simulink model "plant_examples"  (R2023b)
settings: Solver=VariableStepAuto  StartTime=0.0  StopTime=10.0  RelTol=1e-3
undefined symbols (not defined in the file or in its folder): param, x0
libraries: fl_lib x40, nesl_utility x18, simulink x8
(part 3 of 3)

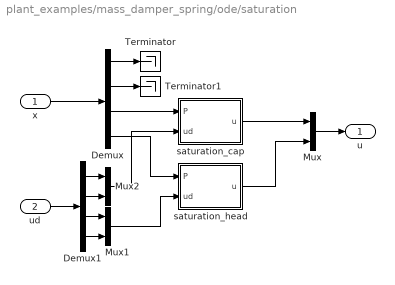
== system plant_examples/mass_damper_spring/ode/saturation ==
  x : Inport  PortDimensions=param.xdim
  ud : Inport  Port=2  PortDimensions=param.udim
  Demux : Demux
  Demux1 : Demux
  Mux : Mux  Inputs=2
  Mux1 : Mux  Inputs=2
  Mux2 : Mux  Inputs=2
  Terminator : Terminator
  Terminator1 : Terminator
  saturation_cap : Subsystem
  saturation_head : Subsystem
  u : Outport
  wires:
  x/1 -> Demux/1
  Demux/3 -> saturation_cap/1(P)
  Demux/4 -> saturation_head/1(P)
  Demux/1 -> Terminator/1
  Demux/2 -> Terminator1/1
  saturation_cap/1(u) -> Mux/1
  saturation_head/1(u) -> Mux/2
  Mux/1 -> u/1
  ud/1 -> Demux1/1
  Demux1/4 -> Mux1/2
  Demux1/3 -> Mux1/1
  Demux1/1 -> Mux2/1
  Demux1/2 -> Mux2/2
  Mux2/1 -> saturation_cap/2(ud)
  Mux1/1 -> saturation_head/2(ud)

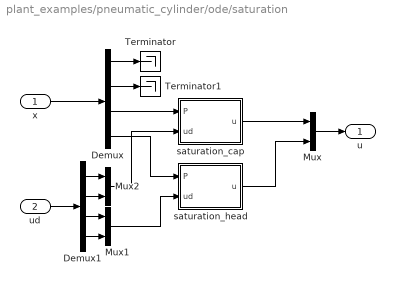
== system plant_examples/pneumatic_cylinder/ode/saturation ==
  x : Inport  PortDimensions=param.xdim
  ud : Inport  Port=2  PortDimensions=param.udim
  Demux : Demux
  Demux1 : Demux
  Mux : Mux  Inputs=2
  Mux1 : Mux  Inputs=2
  Mux2 : Mux  Inputs=2
  Terminator : Terminator
  Terminator1 : Terminator
  saturation_cap : Subsystem
  saturation_head : Subsystem
  u : Outport
  wires:
  x/1 -> Demux/1
  Demux/3 -> saturation_cap/1(P)
  Demux/4 -> saturation_head/1(P)
  Demux/1 -> Terminator/1
  Demux/2 -> Terminator1/1
  saturation_cap/1(u) -> Mux/1
  saturation_head/1(u) -> Mux/2
  Mux/1 -> u/1
  ud/1 -> Demux1/1
  Demux1/4 -> Mux1/2
  Demux1/3 -> Mux1/1
  Demux1/1 -> Mux2/1
  Demux1/2 -> Mux2/2
  Mux2/1 -> saturation_cap/2(ud)
  Mux1/1 -> saturation_head/2(ud)

== system plant_examples/pneumatic_cylinder/simscape/Vctube ==
  Ta : fl_lib/Thermal/Thermal Sources/Temperature Source  temperature=param.Ta K
  Vctube : fl_lib/Gas/Elements/Constant Volume Chamber (G)  volume=param.Vctube m^3  num_ports=foundation.enum.num_ports.one  area_A=0.01 m^2  area_B=0.01 m^2  area_C=0.01 m^2  area_D=0.01 m^2  p_I_specify=on  p_I_priority=High  p_I=x0(3) Pa  p_I_nominal_specify=off  p_I_nominal_unit=MPa  p_I_nominal_value=1  T_I_specify=off  T_I_priority=High  T_I=293.15 K  T_I_nominal_specify=off  T_I_nominal_unit=K  T_I_nominal_value=1  rho_I_specify=off  rho_I_priority=None  rho_I=1.2 kg/m^3  rho_I_nominal_specify=off  rho_I_nominal_unit=kg/m^3  rho_I_nominal_value=1
      settings: InternalSimscapePortConfiguration="{\"Bottom\":[],\"Left\":[{\"id\":\"A\",\"label\":\"A\",\"type\":\"foundation.gas.gas\"},{\"id\":\"H\",\"label\":\"H\",\"type\":\"foundation.thermal.thermal\"}],\"Right\":[],\"Top\":[]}"
  A : PMIOPort  Side=Left
  B : PMIOPort  Port=2  Side=Right
  connections:
  A/RConn1 -- B/RConn1 -- Vctube/LConn1
  Ta/LConn1 -- Vctube/LConn2

== system plant_examples/pneumatic_cylinder/simscape/Vhtube ==
  Ta : fl_lib/Thermal/Thermal Sources/Temperature Source  temperature=param.Ta K
  Vhtube : fl_lib/Gas/Elements/Constant Volume Chamber (G)  volume=param.Vhtube m^3  num_ports=foundation.enum.num_ports.one  area_A=0.01 m^2  area_B=0.01 m^2  area_C=0.01 m^2  area_D=0.01 m^2  p_I_specify=on  p_I_priority=High  p_I=x0(4) Pa  p_I_nominal_specify=off  p_I_nominal_unit=MPa  p_I_nominal_value=1  T_I_specify=off  T_I_priority=High  T_I=293.15 K  T_I_nominal_specify=off  T_I_nominal_unit=K  T_I_nominal_value=1  rho_I_specify=off  rho_I_priority=None  rho_I=1.2 kg/m^3  rho_I_nominal_specify=off  rho_I_nominal_unit=kg/m^3  rho_I_nominal_value=1
      settings: InternalSimscapePortConfiguration="{\"Bottom\":[],\"Left\":[{\"id\":\"A\",\"label\":\"A\",\"type\":\"foundation.gas.gas\"},{\"id\":\"H\",\"label\":\"H\",\"type\":\"foundation.thermal.thermal\"}],\"Right\":[],\"Top\":[]}"
  A : PMIOPort  Side=Left
  B : PMIOPort  Port=2  Side=Right
  connections:
  A/RConn1 -- Vhtube/LConn1 -- B/RConn1
  Ta/LConn1 -- Vhtube/LConn2

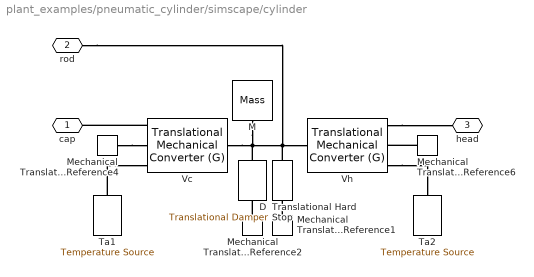
== system plant_examples/pneumatic_cylinder/simscape/cylinder ==
  D : fl_lib/Mechanical/Translational Elements/Translational Damper  D=param.D N*s/m  v_specify=off  v_priority=None  v=0 m/s  v_nominal_specify=off  v_nominal_unit=m/s  v_nominal_value=1  f_specify=off  f_priority=None  f=0 N  f_nominal_specify=off  f_nominal_unit=N  f_nominal_value=1
  M : fl_lib/Mechanical/Translational Elements/Mass  mass=param.M kg  num_ports=foundation.enum.numPorts2.one  v_specify=off  v_priority=High  v=0 m/s  v_nominal_specify=off  v_nominal_unit=m/s  v_nominal_value=1  f_specify=off  f_priority=None  f=0 N  f_nominal_specify=off  f_nominal_unit=N  f_nominal_value=1
  Mechanical Translational Reference{1..2,4,6} (4 alike) : fl_lib/Mechanical/Translational Elements/Mechanical Translational Reference
  Ta1 : fl_lib/Thermal/Thermal Sources/Temperature Source  temperature=param.Ta K
  Ta2 : fl_lib/Thermal/Thermal Sources/Temperature Source  temperature=param.Ta K
  Translational Hard Stop : fl_lib/Mechanical/Translational Elements/Translational Hard Stop  upper_bnd=0.5*param.L m  lower_bnd=-0.5*param.L m  model=simscape.enum.hardstop.fulldamped  stiff_up=1e6 N/m  stiff_low=1e6 N/m  D_up=150 N*s/m  D_low=150 N*s/m  transition=0.1 mm  coeff_rest=0.7  v_tol=0.001 m/s  f_tol=0.001 N  v_specify=off  v_priority=None  v=0 m/s  v_nominal_specify=off  v_nominal_unit=m/s  v_nominal_value=1  f_specify=off  f_priority=None  f=0 N  f_nominal_specify=off  f_nominal_unit=N  f_nominal_value=1  x_specify=on  x_priority=High  x=x0(1) m  x_nominal_specify=off  x_nominal_unit=m  x_nominal_value=1  M_specify=off  M_priority=None  M=0
  Vc : fl_lib/Gas/Elements/Translational Mechanical Converter (G)  mech_orientation=foundation.enum.MechOrientationTranslational.Positive  displacement_spec=foundation.enum.DisplacementSpec.Calculate  length_init=x0(1)+0.5*param.L m  interface_area=param.Ac m^2  dead_volume=param.Vc0 m^3  area_A=0.01 m^2  environment_spec=foundation.enum.pressure_spec.atmospheric  environment_pressure=0.101325 MPa  p_I_specify=on  p_I_priority=High  p_I=x0(3) Pa  p_I_nominal_specify=off  p_I_nominal_unit=MPa  p_I_nominal_value=1  T_I_specify=off  T_I_priority=High  T_I=293.15 K  T_I_nominal_specify=off  T_I_nominal_unit=K  T_I_nominal_value=1  rho_I_specify=off  rho_I_priority=None  rho_I=1.2 kg/m^3  rho_I_nominal_specify=off  rho_I_nominal_unit=kg/m^3  rho_I_nominal_value=1
      settings: InternalSimscapePortConfiguration="{\"Bottom\":[],\"Left\":[{\"id\":\"A\",\"label\":\"A\",\"type\":\"foundation.gas.gas\"},{\"id\":\"C\",\"label\":\"C\",\"type\":\"foundation.mechanical.translational.translational\"},{\"id\":\"H\",\"label\":\"H\",\"type\":\"foundation.thermal.thermal\"}],\"Right\":[{\"id\":\"R\",\"label\":\"R\",\"type\":\"foundation.mechanical.translational.translational\"}],\"Top\":[]}"
  Vh : fl_lib/Gas/Elements/Translational Mechanical Converter (G)  mech_orientation=foundation.enum.MechOrientationTranslational.Negative  displacement_spec=foundation.enum.DisplacementSpec.Calculate  length_init=x0(1)-0.5*param.L m  interface_area=param.Ah m^2  dead_volume=param.Vh0 m^3  area_A=0.01 m^2  environment_spec=foundation.enum.pressure_spec.atmospheric  environment_pressure=0.101325 MPa  p_I_specify=on  p_I_priority=High  p_I=x0(4) Pa  p_I_nominal_specify=off  p_I_nominal_unit=MPa  p_I_nominal_value=1  T_I_specify=off  T_I_priority=High  T_I=293.15 K  T_I_nominal_specify=off  T_I_nominal_unit=K  T_I_nominal_value=1  rho_I_specify=off  rho_I_priority=None  rho_I=1.2 kg/m^3  rho_I_nominal_specify=off  rho_I_nominal_unit=kg/m^3  rho_I_nominal_value=1
      settings: InternalSimscapePortConfiguration="{\"Bottom\":[],\"Left\":[{\"id\":\"A\",\"label\":\"A\",\"type\":\"foundation.gas.gas\"},{\"id\":\"C\",\"label\":\"C\",\"type\":\"foundation.mechanical.translational.translational\"},{\"id\":\"H\",\"label\":\"H\",\"type\":\"foundation.thermal.thermal\"}],\"Right\":[{\"id\":\"R\",\"label\":\"R\",\"type\":\"foundation.mechanical.translational.translational\"}],\"Top\":[]}"
  cap : PMIOPort  Side=Left
  rod : PMIOPort  Port=2  Side=Left
  head : PMIOPort  Port=3  Side=Right
  connections:
  Mechanical Translational Reference4/LConn1 -- Vc/LConn2
  Mechanical Translational Reference6/LConn1 -- Vh/LConn2
  Vh/LConn1 -- head/RConn1
  Mechanical Translational Reference2/LConn1 -- D/RConn1
  Vc/RConn1 -- rod/RConn1 -- Translational Hard Stop/LConn1 -- Vh/RConn1 -- M/LConn1 -- D/LConn1
  Mechanical Translational Reference1/LConn1 -- Translational Hard Stop/RConn1
  Vc/LConn1 -- cap/RConn1
  Ta1/LConn1 -- Vc/LConn3
  Vh/LConn3 -- Ta2/LConn1

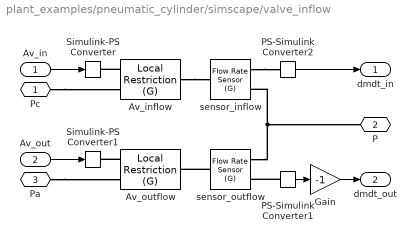
== system plant_examples/pneumatic_cylinder/simscape/valve_inflow ==
  Av_in : Inport
  Av_out : Inport  Port=2
  Av_inflow : fl_lib/Gas/Elements/Local Restriction (G)  restriction_type=foundation.enum.restriction_type.variable  restriction_area=1e-3 m^2  min_area=eps m^2  max_area=param.Av m^2  area=0.01 m^2  Cd=0.8975  B_lam=0.999
      settings: InternalSimscapePortConfiguration="{\"Bottom\":[],\"Left\":[{\"id\":\"A\",\"label\":\"A\",\"type\":\"foundation.gas.gas\"},{\"id\":\"area_in\",\"label\":\"AR\",\"type\":\"input\"}],\"Right\":[{\"id\":\"B\",\"label\":\"B\",\"type\":\"foundation.gas.gas\"}],\"Top\":[]}"
  Av_outflow : fl_lib/Gas/Elements/Local Restriction (G)  restriction_type=foundation.enum.restriction_type.variable  restriction_area=1e-3 m^2  min_area=eps m^2  max_area=param.Av m^2  area=0.01 m^2  Cd=0.8975  B_lam=0.999
      settings: InternalSimscapePortConfiguration="{\"Bottom\":[],\"Left\":[{\"id\":\"A\",\"label\":\"A\",\"type\":\"foundation.gas.gas\"},{\"id\":\"area_in\",\"label\":\"AR\",\"type\":\"input\"}],\"Right\":[{\"id\":\"B\",\"label\":\"B\",\"type\":\"foundation.gas.gas\"}],\"Top\":[]}"
  Gain : Gain  Gain=-1
  PS-Simulink Converter1 : nesl_utility/PS-Simulink Converter  PhysicalDomain=network_engine_domain  SubClassName=ps_output  LeftPortType=input  RightPortType=output  PseudoPeriodic=off  Frequencies=[]  VectorFormat=inherit  Unit=inherit  AffineConversion=off
  PS-Simulink Converter2 : nesl_utility/PS-Simulink Converter  PhysicalDomain=network_engine_domain  SubClassName=ps_output  LeftPortType=input  RightPortType=output  PseudoPeriodic=off  Frequencies=[]  VectorFormat=inherit  Unit=inherit  AffineConversion=off
  Simulink-PS Converter : nesl_utility/Simulink-PS Converter  PhysicalDomain=network_engine_domain  SubClassName=ps_input  LeftPortType=input  RightPortType=output  PseudoPeriodic=off  Frequencies=[]  NoiseDistribution=none  NoiseParameters=[]  Unit=1  AffineConversion=off  FilteringAndDerivatives=provide  SimscapeFilterOrder=1  InputFilterTimeConstant=0.001  UdotUserProvided=0
  Simulink-PS Converter1 : nesl_utility/Simulink-PS Converter  PhysicalDomain=network_engine_domain  SubClassName=ps_input  LeftPortType=input  RightPortType=output  PseudoPeriodic=off  Frequencies=[]  NoiseDistribution=none  NoiseParameters=[]  Unit=1  AffineConversion=off  FilteringAndDerivatives=provide  SimscapeFilterOrder=1  InputFilterTimeConstant=0.001  UdotUserProvided=0
  sensor_inflow : fl_lib/Gas/Sensors/Flow Rate Sensor (G)  mass_flow_measure=true  volumetric_flow_measure=false  volumetric_flow_conditions=foundation.enum.volumetric_flow_conditions.actual  p_std=0.101325 MPa  T_std=20 degC  energy_flow_measure=false
      settings: InternalSimscapePortConfiguration="{\"Bottom\":[],\"Left\":[{\"id\":\"A\",\"label\":\"A\",\"type\":\"foundation.gas.gas\"}],\"Right\":[{\"id\":\"B\",\"label\":\"B\",\"type\":\"foundation.gas.gas\"},{\"id\":\"M\",\"label\":\"M\",\"type\":\"output\"}],\"Top\":[]}"
  sensor_outflow : fl_lib/Gas/Sensors/Flow Rate Sensor (G)  mass_flow_measure=true  volumetric_flow_measure=false  volumetric_flow_conditions=foundation.enum.volumetric_flow_conditions.actual  p_std=0.101325 MPa  T_std=20 degC  energy_flow_measure=false
      settings: InternalSimscapePortConfiguration="{\"Bottom\":[],\"Left\":[{\"id\":\"A\",\"label\":\"A\",\"type\":\"foundation.gas.gas\"}],\"Right\":[{\"id\":\"B\",\"label\":\"B\",\"type\":\"foundation.gas.gas\"},{\"id\":\"M\",\"label\":\"M\",\"type\":\"output\"}],\"Top\":[]}"
  Pc : PMIOPort  Side=Left
  P : PMIOPort  Port=2  Side=Right
  Pa : PMIOPort  Port=3  Side=Right
  dmdt_in : Outport
  dmdt_out : Outport  Port=2
  wires:
  Av_in/1 -> Simulink-PS Converter/1
  Av_out/1 -> Simulink-PS Converter1/1
  PS-Simulink Converter2/1 -> dmdt_in/1
  PS-Simulink Converter1/1 -> Gain/1
  Gain/1 -> dmdt_out/1
  connections:
  Av_inflow/RConn1 -- sensor_inflow/LConn1
  Pc/RConn1 -- Av_inflow/LConn1
  Av_inflow/LConn2 -- Simulink-PS Converter/RConn1
  Pa/RConn1 -- Av_outflow/LConn1
  sensor_outflow/RConn1 -- sensor_inflow/RConn1 -- P/RConn1
  Av_outflow/LConn2 -- Simulink-PS Converter1/RConn1
  sensor_outflow/LConn1 -- Av_outflow/RConn1
  sensor_inflow/RConn2 -- PS-Simulink Converter2/LConn1
  PS-Simulink Converter1/LConn1 -- sensor_outflow/RConn2

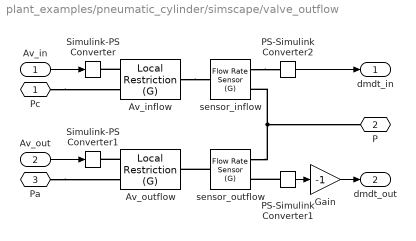
== system plant_examples/pneumatic_cylinder/simscape/valve_outflow ==
  Av_in : Inport
  Av_out : Inport  Port=2
  Av_inflow : fl_lib/Gas/Elements/Local Restriction (G)  restriction_type=foundation.enum.restriction_type.variable  restriction_area=1e-3 m^2  min_area=eps m^2  max_area=param.Av m^2  area=0.01 m^2  Cd=0.8975  B_lam=0.999
      settings: InternalSimscapePortConfiguration="{\"Bottom\":[],\"Left\":[{\"id\":\"A\",\"label\":\"A\",\"type\":\"foundation.gas.gas\"},{\"id\":\"area_in\",\"label\":\"AR\",\"type\":\"input\"}],\"Right\":[{\"id\":\"B\",\"label\":\"B\",\"type\":\"foundation.gas.gas\"}],\"Top\":[]}"
  Av_outflow : fl_lib/Gas/Elements/Local Restriction (G)  restriction_type=foundation.enum.restriction_type.variable  restriction_area=1e-3 m^2  min_area=eps m^2  max_area=param.Av m^2  area=0.01 m^2  Cd=0.8975  B_lam=0.999
      settings: InternalSimscapePortConfiguration="{\"Bottom\":[],\"Left\":[{\"id\":\"A\",\"label\":\"A\",\"type\":\"foundation.gas.gas\"},{\"id\":\"area_in\",\"label\":\"AR\",\"type\":\"input\"}],\"Right\":[{\"id\":\"B\",\"label\":\"B\",\"type\":\"foundation.gas.gas\"}],\"Top\":[]}"
  Gain : Gain  Gain=-1
  PS-Simulink Converter1 : nesl_utility/PS-Simulink Converter  PhysicalDomain=network_engine_domain  SubClassName=ps_output  LeftPortType=input  RightPortType=output  PseudoPeriodic=off  Frequencies=[]  VectorFormat=inherit  Unit=inherit  AffineConversion=off
  PS-Simulink Converter2 : nesl_utility/PS-Simulink Converter  PhysicalDomain=network_engine_domain  SubClassName=ps_output  LeftPortType=input  RightPortType=output  PseudoPeriodic=off  Frequencies=[]  VectorFormat=inherit  Unit=inherit  AffineConversion=off
  Simulink-PS Converter : nesl_utility/Simulink-PS Converter  PhysicalDomain=network_engine_domain  SubClassName=ps_input  LeftPortType=input  RightPortType=output  PseudoPeriodic=off  Frequencies=[]  NoiseDistribution=none  NoiseParameters=[]  Unit=1  AffineConversion=off  FilteringAndDerivatives=provide  SimscapeFilterOrder=1  InputFilterTimeConstant=0.001  UdotUserProvided=0
  Simulink-PS Converter1 : nesl_utility/Simulink-PS Converter  PhysicalDomain=network_engine_domain  SubClassName=ps_input  LeftPortType=input  RightPortType=output  PseudoPeriodic=off  Frequencies=[]  NoiseDistribution=none  NoiseParameters=[]  Unit=1  AffineConversion=off  FilteringAndDerivatives=provide  SimscapeFilterOrder=1  InputFilterTimeConstant=0.001  UdotUserProvided=0
  sensor_inflow : fl_lib/Gas/Sensors/Flow Rate Sensor (G)  mass_flow_measure=true  volumetric_flow_measure=false  volumetric_flow_conditions=foundation.enum.volumetric_flow_conditions.actual  p_std=0.101325 MPa  T_std=20 degC  energy_flow_measure=false
      settings: InternalSimscapePortConfiguration="{\"Bottom\":[],\"Left\":[{\"id\":\"A\",\"label\":\"A\",\"type\":\"foundation.gas.gas\"}],\"Right\":[{\"id\":\"B\",\"label\":\"B\",\"type\":\"foundation.gas.gas\"},{\"id\":\"M\",\"label\":\"M\",\"type\":\"output\"}],\"Top\":[]}"
  sensor_outflow : fl_lib/Gas/Sensors/Flow Rate Sensor (G)  mass_flow_measure=true  volumetric_flow_measure=false  volumetric_flow_conditions=foundation.enum.volumetric_flow_conditions.actual  p_std=0.101325 MPa  T_std=20 degC  energy_flow_measure=false
      settings: InternalSimscapePortConfiguration="{\"Bottom\":[],\"Left\":[{\"id\":\"A\",\"label\":\"A\",\"type\":\"foundation.gas.gas\"}],\"Right\":[{\"id\":\"B\",\"label\":\"B\",\"type\":\"foundation.gas.gas\"},{\"id\":\"M\",\"label\":\"M\",\"type\":\"output\"}],\"Top\":[]}"
  Pc : PMIOPort  Side=Left
  P : PMIOPort  Port=2  Side=Right
  Pa : PMIOPort  Port=3  Side=Right
  dmdt_in : Outport
  dmdt_out : Outport  Port=2
  wires:
  Av_in/1 -> Simulink-PS Converter/1
  Av_out/1 -> Simulink-PS Converter1/1
  PS-Simulink Converter2/1 -> dmdt_in/1
  PS-Simulink Converter1/1 -> Gain/1
  Gain/1 -> dmdt_out/1
  connections:
  Av_inflow/RConn1 -- sensor_inflow/LConn1
  Pc/RConn1 -- Av_inflow/LConn1
  Av_inflow/LConn2 -- Simulink-PS Converter/RConn1
  Pa/RConn1 -- Av_outflow/LConn1
  sensor_outflow/RConn1 -- P/RConn1 -- sensor_inflow/RConn1
  Av_outflow/LConn2 -- Simulink-PS Converter1/RConn1
  sensor_outflow/LConn1 -- Av_outflow/RConn1
  sensor_inflow/RConn2 -- PS-Simulink Converter2/LConn1
  PS-Simulink Converter1/LConn1 -- sensor_outflow/RConn2

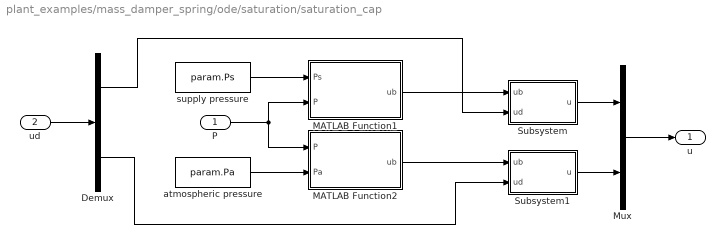
== system plant_examples/mass_damper_spring/ode/saturation/saturation_cap ==
  P : Inport
  ud : Inport  Port=2
  Demux : Demux  Outputs=2
  MATLAB Function1 : MATLAB Function  TreatAsAtomicUnit=on
  MATLAB Function2 : MATLAB Function  TreatAsAtomicUnit=on
  Mux : Mux  Inputs=2
  Subsystem : Subsystem
  Subsystem1 : Subsystem
  atmospheric pressure : Constant  Value=param.Pa
  supply pressure : Constant  Value=param.Ps
  u : Outport
  wires:
  ud/1 -> Demux/1
  Mux/1 -> u/1
  supply pressure/1 -> MATLAB Function1/1(Ps)
  P/1 -> MATLAB Function1/2(P), MATLAB Function2/1(P)
  atmospheric pressure/1 -> MATLAB Function2/2(Pa)
  MATLAB Function1/1(ub) -> Subsystem/1(ub)
  MATLAB Function2/1(ub) -> Subsystem1/1(ub)
  Demux/1 -> Subsystem/2(ud)
  Demux/2 -> Subsystem1/2(ud)
  Subsystem/1(u) -> Mux/1
  Subsystem1/1(u) -> Mux/2

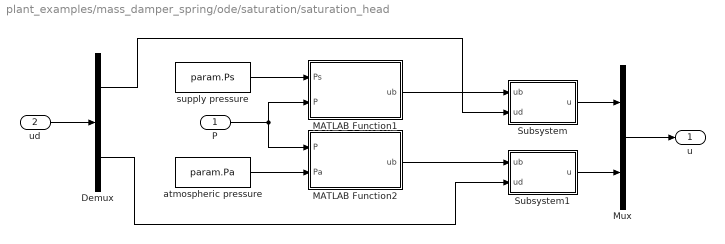
== system plant_examples/mass_damper_spring/ode/saturation/saturation_head ==
  P : Inport
  ud : Inport  Port=2
  Demux : Demux  Outputs=2
  MATLAB Function1 : MATLAB Function  TreatAsAtomicUnit=on
  MATLAB Function2 : MATLAB Function  TreatAsAtomicUnit=on
  Mux : Mux  Inputs=2
  Subsystem : Subsystem
  Subsystem1 : Subsystem
  atmospheric pressure : Constant  Value=param.Pa
  supply pressure : Constant  Value=param.Ps
  u : Outport
  wires:
  ud/1 -> Demux/1
  Mux/1 -> u/1
  supply pressure/1 -> MATLAB Function1/1(Ps)
  P/1 -> MATLAB Function1/2(P), MATLAB Function2/1(P)
  atmospheric pressure/1 -> MATLAB Function2/2(Pa)
  MATLAB Function1/1(ub) -> Subsystem/1(ub)
  MATLAB Function2/1(ub) -> Subsystem1/1(ub)
  Demux/1 -> Subsystem/2(ud)
  Demux/2 -> Subsystem1/2(ud)
  Subsystem/1(u) -> Mux/1
  Subsystem1/1(u) -> Mux/2

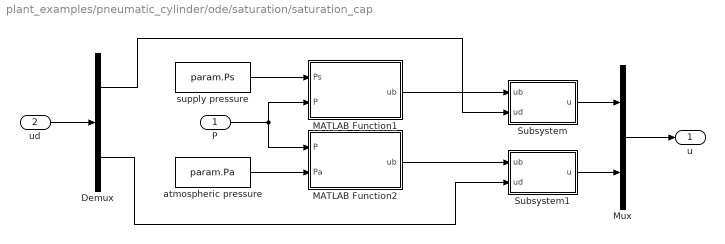
== system plant_examples/pneumatic_cylinder/ode/saturation/saturation_cap ==
  P : Inport
  ud : Inport  Port=2
  Demux : Demux  Outputs=2
  MATLAB Function1 : MATLAB Function  TreatAsAtomicUnit=on
  MATLAB Function2 : MATLAB Function  TreatAsAtomicUnit=on
  Mux : Mux  Inputs=2
  Subsystem : Subsystem
  Subsystem1 : Subsystem
  atmospheric pressure : Constant  Value=param.Pa
  supply pressure : Constant  Value=param.Ps
  u : Outport
  wires:
  ud/1 -> Demux/1
  Mux/1 -> u/1
  supply pressure/1 -> MATLAB Function1/1(Ps)
  P/1 -> MATLAB Function1/2(P), MATLAB Function2/1(P)
  atmospheric pressure/1 -> MATLAB Function2/2(Pa)
  MATLAB Function1/1(ub) -> Subsystem/1(ub)
  MATLAB Function2/1(ub) -> Subsystem1/1(ub)
  Demux/1 -> Subsystem/2(ud)
  Demux/2 -> Subsystem1/2(ud)
  Subsystem/1(u) -> Mux/1
  Subsystem1/1(u) -> Mux/2

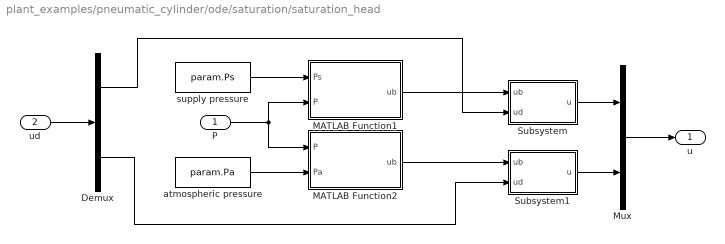
== system plant_examples/pneumatic_cylinder/ode/saturation/saturation_head ==
  P : Inport
  ud : Inport  Port=2
  Demux : Demux  Outputs=2
  MATLAB Function1 : MATLAB Function  TreatAsAtomicUnit=on
  MATLAB Function2 : MATLAB Function  TreatAsAtomicUnit=on
  Mux : Mux  Inputs=2
  Subsystem : Subsystem
  Subsystem1 : Subsystem
  atmospheric pressure : Constant  Value=param.Pa
  supply pressure : Constant  Value=param.Ps
  u : Outport
  wires:
  ud/1 -> Demux/1
  Mux/1 -> u/1
  supply pressure/1 -> MATLAB Function1/1(Ps)
  P/1 -> MATLAB Function1/2(P), MATLAB Function2/1(P)
  atmospheric pressure/1 -> MATLAB Function2/2(Pa)
  MATLAB Function1/1(ub) -> Subsystem/1(ub)
  MATLAB Function2/1(ub) -> Subsystem1/1(ub)
  Demux/1 -> Subsystem/2(ud)
  Demux/2 -> Subsystem1/2(ud)
  Subsystem/1(u) -> Mux/1
  Subsystem1/1(u) -> Mux/2

== system plant_examples/mass_damper_spring/ode/saturation/saturation_cap/Subsystem ==
  ub : Inport
  ud : Inport  Port=2
  Constant : Constant  Value=0
  Max : MinMax  Function=max  Inputs=2
  Min : MinMax  Inputs=2
  Saturation Dynamic : simulink/Discontinuities/Saturation Dynamic  OutMin=[]  OutMax=[]  OutDataTypeStr=Inherit: Same as second input  OutDataType=fixdt(1, 16)  OutScaling=2^-10  DoSatur=off
  u : Outport
  wires:
  Min/1 -> Saturation Dynamic/3
  ud/1 -> Saturation Dynamic/2
  Constant/1 -> Max/2, Min/2
  Max/1 -> Saturation Dynamic/1
  Saturation Dynamic/1 -> u/1
  ub/1 -> Min/1, Max/1

== system plant_examples/mass_damper_spring/ode/saturation/saturation_cap/Subsystem1 ==
  ub : Inport
  ud : Inport  Port=2
  Constant : Constant  Value=0
  Max : MinMax  Function=max  Inputs=2
  Min : MinMax  Inputs=2
  Saturation Dynamic : simulink/Discontinuities/Saturation Dynamic  OutMin=[]  OutMax=[]  OutDataTypeStr=Inherit: Same as second input  OutDataType=fixdt(1, 16)  OutScaling=2^-10  DoSatur=off
  u : Outport
  wires:
  ub/1 -> Max/1, Min/1
  Saturation Dynamic/1 -> u/1
  Max/1 -> Saturation Dynamic/1
  Constant/1 -> Min/2, Max/2
  ud/1 -> Saturation Dynamic/2
  Min/1 -> Saturation Dynamic/3

== system plant_examples/mass_damper_spring/ode/saturation/saturation_head/Subsystem ==
  ub : Inport
  ud : Inport  Port=2
  Constant : Constant  Value=0
  Max : MinMax  Function=max  Inputs=2
  Min : MinMax  Inputs=2
  Saturation Dynamic : simulink/Discontinuities/Saturation Dynamic  OutMin=[]  OutMax=[]  OutDataTypeStr=Inherit: Same as second input  OutDataType=fixdt(1, 16)  OutScaling=2^-10  DoSatur=off
  u : Outport
  wires:
  Min/1 -> Saturation Dynamic/3
  ud/1 -> Saturation Dynamic/2
  Constant/1 -> Max/2, Min/2
  Max/1 -> Saturation Dynamic/1
  Saturation Dynamic/1 -> u/1
  ub/1 -> Min/1, Max/1

== system plant_examples/mass_damper_spring/ode/saturation/saturation_head/Subsystem1 ==
  ub : Inport
  ud : Inport  Port=2
  Constant : Constant  Value=0
  Max : MinMax  Function=max  Inputs=2
  Min : MinMax  Inputs=2
  Saturation Dynamic : simulink/Discontinuities/Saturation Dynamic  OutMin=[]  OutMax=[]  OutDataTypeStr=Inherit: Same as second input  OutDataType=fixdt(1, 16)  OutScaling=2^-10  DoSatur=off
  u : Outport
  wires:
  ub/1 -> Max/1, Min/1
  Saturation Dynamic/1 -> u/1
  Max/1 -> Saturation Dynamic/1
  Constant/1 -> Min/2, Max/2
  ud/1 -> Saturation Dynamic/2
  Min/1 -> Saturation Dynamic/3

== system plant_examples/pneumatic_cylinder/ode/saturation/saturation_cap/Subsystem ==
  ub : Inport
  ud : Inport  Port=2
  Constant : Constant  Value=0
  Max : MinMax  Function=max  Inputs=2
  Min : MinMax  Inputs=2
  Saturation Dynamic : simulink/Discontinuities/Saturation Dynamic  OutMin=[]  OutMax=[]  OutDataTypeStr=Inherit: Same as second input  OutDataType=fixdt(1, 16)  OutScaling=2^-10  DoSatur=off
  u : Outport
  wires:
  Min/1 -> Saturation Dynamic/3
  ud/1 -> Saturation Dynamic/2
  Constant/1 -> Max/2, Min/2
  Max/1 -> Saturation Dynamic/1
  Saturation Dynamic/1 -> u/1
  ub/1 -> Min/1, Max/1

== system plant_examples/pneumatic_cylinder/ode/saturation/saturation_cap/Subsystem1 ==
  ub : Inport
  ud : Inport  Port=2
  Constant : Constant  Value=0
  Max : MinMax  Function=max  Inputs=2
  Min : MinMax  Inputs=2
  Saturation Dynamic : simulink/Discontinuities/Saturation Dynamic  OutMin=[]  OutMax=[]  OutDataTypeStr=Inherit: Same as second input  OutDataType=fixdt(1, 16)  OutScaling=2^-10  DoSatur=off
  u : Outport
  wires:
  ub/1 -> Max/1, Min/1
  Saturation Dynamic/1 -> u/1
  Max/1 -> Saturation Dynamic/1
  Constant/1 -> Min/2, Max/2
  ud/1 -> Saturation Dynamic/2
  Min/1 -> Saturation Dynamic/3

== system plant_examples/pneumatic_cylinder/ode/saturation/saturation_head/Subsystem ==
  ub : Inport
  ud : Inport  Port=2
  Constant : Constant  Value=0
  Max : MinMax  Function=max  Inputs=2
  Min : MinMax  Inputs=2
  Saturation Dynamic : simulink/Discontinuities/Saturation Dynamic  OutMin=[]  OutMax=[]  OutDataTypeStr=Inherit: Same as second input  OutDataType=fixdt(1, 16)  OutScaling=2^-10  DoSatur=off
  u : Outport
  wires:
  Min/1 -> Saturation Dynamic/3
  ud/1 -> Saturation Dynamic/2
  Constant/1 -> Max/2, Min/2
  Max/1 -> Saturation Dynamic/1
  Saturation Dynamic/1 -> u/1
  ub/1 -> Min/1, Max/1

== system plant_examples/pneumatic_cylinder/ode/saturation/saturation_head/Subsystem1 ==
  ub : Inport
  ud : Inport  Port=2
  Constant : Constant  Value=0
  Max : MinMax  Function=max  Inputs=2
  Min : MinMax  Inputs=2
  Saturation Dynamic : simulink/Discontinuities/Saturation Dynamic  OutMin=[]  OutMax=[]  OutDataTypeStr=Inherit: Same as second input  OutDataType=fixdt(1, 16)  OutScaling=2^-10  DoSatur=off
  u : Outport
  wires:
  ub/1 -> Max/1, Min/1
  Saturation Dynamic/1 -> u/1
  Max/1 -> Saturation Dynamic/1
  Constant/1 -> Min/2, Max/2
  ud/1 -> Saturation Dynamic/2
  Min/1 -> Saturation Dynamic/3

== matlab function plant_examples/pneumatic_cylinder/ode/MATLAB Function ==
  data: x input size=param.xdim; u input size=param.udim; dxdt output size=param.xdim; param parameter
function dxdt = ode(x,u,param)
    dxdt = plant_ode(0,x,u,param);
end

== matlab function plant_examples/pneumatic_cylinder/ode/saturation/saturation_cap/MATLAB Function2 ==
  data: P input; Pa input; ub output; param parameter
function ub = outflow(P,Pa,param)
    ub = input_constraint(P,Pa,param);
end

== matlab function plant_examples/pneumatic_cylinder/ode/saturation/saturation_head/MATLAB Function1 ==
  data: Ps input; P input; ub output; param parameter
function ub = inflow(Ps,P,param)
    ub = input_constraint(Ps,P,param);
end

== matlab function plant_examples/pneumatic_cylinder/ode/saturation/saturation_head/MATLAB Function2 ==
  data: P input; Pa input; ub output; param parameter
function ub = outflow(P,Pa,param)
    ub = input_constraint(P,Pa,param);
end

== matlab function plant_examples/mass_damper_spring/ode/MATLAB Function ==
  data: x input size=param.xdim; u input size=param.udim; dxdt output size=param.xdim; param parameter
function dxdt = ode(x,u,param)
    dxdt = plant_ode(0,x,u,param);
end

== matlab function plant_examples/mass_damper_spring/ode/saturation/saturation_cap/MATLAB Function1 ==
  data: Ps input; P input; ub output; param parameter
function ub = inflow(Ps,P,param)
    ub = input_constraint(Ps,P,param);
end

== matlab function plant_examples/mass_damper_spring/ode/saturation/saturation_cap/MATLAB Function2 ==
  data: P input; Pa input; ub output; param parameter
function ub = outflow(P,Pa,param)
    ub = input_constraint(P,Pa,param);
end

== matlab function plant_examples/mass_damper_spring/ode/saturation/saturation_head/MATLAB Function1 ==
  data: Ps input; P input; ub output; param parameter
function ub = inflow(Ps,P,param)
    ub = input_constraint(Ps,P,param);
end

== matlab function plant_examples/pneumatic_cylinder/ode/saturation/saturation_cap/MATLAB Function1 ==
  data: Ps input; P input; ub output; param parameter
function ub = inflow(Ps,P,param)
    ub = input_constraint(Ps,P,param);
end

== matlab function plant_examples/mass_damper_spring/ode/saturation/saturation_head/MATLAB Function2 ==
  data: P input; Pa input; ub output; param parameter
function ub = outflow(P,Pa,param)
    ub = input_constraint(P,Pa,param);
end
